simulink library "ESTS_FRIC_SLIP2"  (R2024b)
settings: Solver=VariableStepAuto  StartTime=0.0  StopTime=10.0  RelTol=1e-3
undefined symbols (not defined in the file): ESTS_FRIC_p1_MovAvgCoef_na, ESTS_FRIC_p_TirSatLim_na
libraries: VUT_lib x4
settings Model: Creator=blatak  LastModifiedBy=blatak

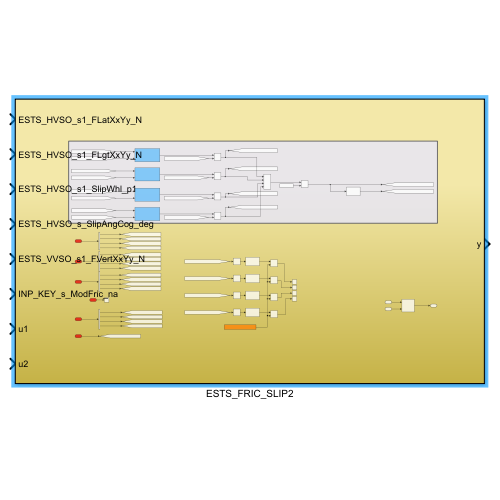
[thumbnail: Simulink's stored preview of the top-level diagram]
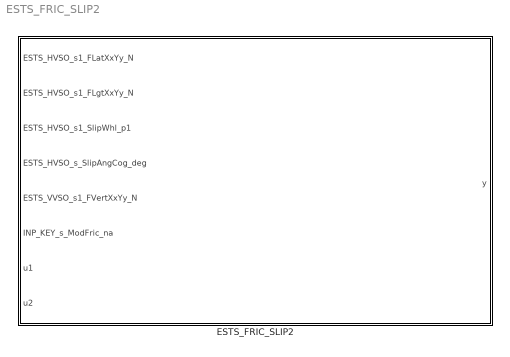
== system ESTS_FRIC_SLIP2 ==
  ESTS_FRIC_SLIP2 : Subsystem

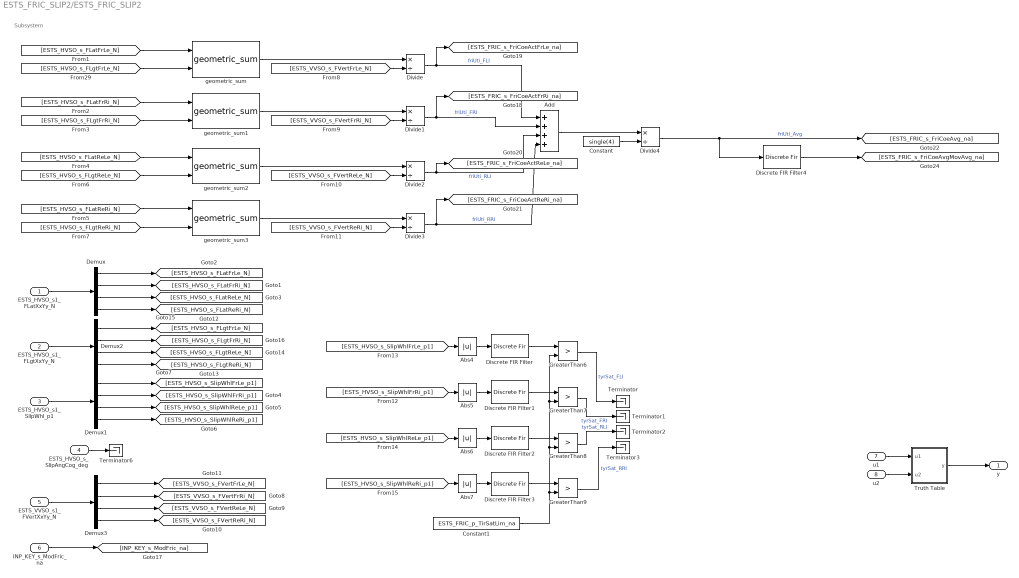
== system ESTS_FRIC_SLIP2/ESTS_FRIC_SLIP2 ==
  note: Subsystem
  ESTS_HVSO_s1_FLatXxYy_N : Inport
  ESTS_HVSO_s1_FLgtXxYy_N : Inport  Port=2
  ESTS_HVSO_s1_SlipWhl_p1 : Inport  Port=3
  ESTS_HVSO_s_SlipAngCog_deg : Inport  Port=4
  ESTS_VVSO_s1_FVertXxYy_N : Inport  Port=5
  INP_KEY_s_ModFric_na : Inport  Port=6
  u1 : Inport  Port=7
  u2 : Inport  Port=8
  Abs{4..7} (4 alike) : Abs  SaturateOnIntegerOverflow=off
  Add : Sum  Inputs=++++
  Constant : Constant  Value=single(4)
  Constant1 : Constant  Value=ESTS_FRIC_p_TirSatLim_na
  Demux{,1..3} (4 alike) : Demux
  Discrete FIR Filter{,1..4} (5 alike) : DiscreteFir  Coefficients=ESTS_FRIC_p1_MovAvgCoef_na
  Divide{,1..4} (5 alike) : Product  Inputs=*/
  GreaterThan{6..9} (4 alike) : RelationalOperator  Operator=>  OutDataTypeStr=boolean  RndMeth=Simplest  InputSameDT=off
  Terminator{,1..3,6} (5 alike) : Terminator
  Truth Table : Truth Table  TreatAsAtomicUnit=on
  geometric_sum{,1..3} (4 alike) : VUT_lib/geometric_sum  SystemSampleTime=-1  VariantActivationTime=update diagram  AllowFlexibleInterface=on  Latency=0  AutoFrameSizeCalculation=off
  y : Outport
  wires:
  [ESTS_HVSO_s_FLatFrLe_N] -> geometric_sum/1
  Divide3/1 -> [ESTS_FRIC_s_FriCoeActReRi_na], Add/4  "friUti_RRI"
  ESTS_VVSO_s1_FVertXxYy_N/1 -> Demux3/1
  GreaterThan7/1 -> Terminator1/1  "tyrSat_FRI"
  [ESTS_VVSO_s_FVertReRi_N] -> Divide3/2
  GreaterThan9/1 -> Terminator3/1  "tyrSat_RRI"
  [ESTS_VVSO_s_FVertFrLe_N] -> Divide/2
  Add/1 -> Divide4/1
  INP_KEY_s_ModFric_na/1 -> [INP_KEY_s_ModFric_na]
  Demux2/4 -> [ESTS_HVSO_s_FLgtReRi_N]
  Demux2/1 -> [ESTS_HVSO_s_FLgtFrLe_N]
  ESTS_HVSO_s1_FLatXxYy_N/1 -> Demux/1
  ESTS_HVSO_s1_SlipWhl_p1/1 -> Demux1/1
  Demux1/4 -> [ESTS_HVSO_s_SlipWhlReRi_p1]
  Demux/2 -> [ESTS_HVSO_s_FLatFrRi_N]
  GreaterThan8/1 -> Terminator2/1  "tyrSat_RLI"
  [ESTS_HVSO_s_SlipWhlReLe_p1] -> Abs6/1
  [ESTS_HVSO_s_SlipWhlFrRi_p1] -> Abs5/1
  [ESTS_HVSO_s_FLatReRi_N] -> geometric_sum3/1
  [ESTS_VVSO_s_FVertReLe_N] -> Divide2/2
  Discrete FIR Filter2/1 -> GreaterThan8/1
  GreaterThan6/1 -> Terminator/1  "tyrSat_FLI"
  Abs6/1 -> Discrete FIR Filter2/1
  ESTS_HVSO_s_SlipAngCog_deg/1 -> Terminator6/1
  [ESTS_HVSO_s_SlipWhlReRi_p1] -> Abs7/1
  Discrete FIR Filter3/1 -> GreaterThan9/1
  Demux/3 -> [ESTS_HVSO_s_FLatReLe_N]
  ESTS_HVSO_s1_FLgtXxYy_N/1 -> Demux2/1
  Demux3/4 -> [ESTS_VVSO_s_FVertReRi_N]
  [ESTS_HVSO_s_SlipWhlFrLe_p1] -> Abs4/1
  Discrete FIR Filter4/1 -> [ESTS_FRIC_s_FriCoeAvgMovAvg_na]
  Divide1/1 -> [ESTS_FRIC_s_FriCoeActFrRi_na], Add/2  "friUti_FRI"
  Constant1/1 -> GreaterThan9/2, GreaterThan8/2, GreaterThan7/2, GreaterThan6/2
  Constant/1 -> Divide4/2
  Demux2/3 -> [ESTS_HVSO_s_FLgtReLe_N]
  Demux3/2 -> [ESTS_VVSO_s_FVertFrRi_N]
  Demux1/2 -> [ESTS_HVSO_s_SlipWhlFrRi_p1]
  [ESTS_HVSO_s_FLatReLe_N] -> geometric_sum2/1
  geometric_sum/1 -> Divide/1
  Demux/4 -> [ESTS_HVSO_s_FLatReRi_N]
  Divide4/1 -> [ESTS_FRIC_s_FriCoeAvg_na], Discrete FIR Filter4/1  "friUti_Avg"
  Discrete FIR Filter/1 -> GreaterThan6/1
  [ESTS_HVSO_s_FLatFrRi_N] -> geometric_sum1/1
  Demux1/3 -> [ESTS_HVSO_s_SlipWhlReLe_p1]
  [ESTS_HVSO_s_FLgtFrLe_N] -> geometric_sum/2
  [ESTS_HVSO_s_FLgtFrRi_N] -> geometric_sum1/2
  Divide2/1 -> [ESTS_FRIC_s_FriCoeActReLe_na], Add/3  "friUti_RLI"
  [ESTS_HVSO_s_FLgtReRi_N] -> geometric_sum3/2
  [ESTS_VVSO_s_FVertFrRi_N] -> Divide1/2
  Demux2/2 -> [ESTS_HVSO_s_FLgtFrRi_N]
  Divide/1 -> Add/1, [ESTS_FRIC_s_FriCoeActFrLe_na]  "friUti_FLI"
  geometric_sum2/1 -> Divide2/1
  [ESTS_HVSO_s_FLgtReLe_N] -> geometric_sum2/2
  Demux1/1 -> [ESTS_HVSO_s_SlipWhlFrLe_p1]
  Demux3/3 -> [ESTS_VVSO_s_FVertReLe_N]
  geometric_sum1/1 -> Divide1/1
  geometric_sum3/1 -> Divide3/1
  Abs4/1 -> Discrete FIR Filter/1
  Discrete FIR Filter1/1 -> GreaterThan7/1
  Demux/1 -> [ESTS_HVSO_s_FLatFrLe_N]
  Abs7/1 -> Discrete FIR Filter3/1
  Demux3/1 -> [ESTS_VVSO_s_FVertFrLe_N]
  Abs5/1 -> Discrete FIR Filter1/1
  u2/1 -> Truth Table/2(u2)
  u1/1 -> Truth Table/1(u1)
  Truth Table/1(y) -> y/1

== matlab function ESTS_FRIC_SLIP2/Truth Table ==
  data: u1 input boolean; y output; u2 input boolean
function y = fcn(u1, u2)

aVarTruthTableCondition_1 = false;
aVarTruthTableCondition_2 = false;


% Example condition 1

aVarTruthTableCondition_1 = logical(u1 >= 0);

% Example condition 2

aVarTruthTableCondition_2 = logical(u ^ 2 <= 1);

if (aVarTruthTableCondition_1 && aVarTruthTableCondition_2)
    aFcnTruthTableAction_1();
elseif (~aVarTruthTableCondition_1 && ~aVarTruthTableCondition_2)
    aFcnTruthTableAction_1();
else % Default
    aFcnTruthTableAction_2();
end

function aFcnTruthTableAction_1()

% Example action 1 called from D1 & D2 column in condition table

y = u;

function aFcnTruthTableAction_2()

% Example action 2 called from D3 column in condition table

y = 1 / u;
